simulink model "PBA3_4"  (R2015a)
settings: Solver=ode45  StartTime=0.0  StopTime=18  MaxStep=0.001  MinStep=0.0001  RelTol=1e-3
values from neighbouring files (symbols this model uses):
  c = 0.08    [Bicycle_whipple.m]    (also in PBA3_2_script.m = 0.1; PBA3_4_script.m = 0.1)
  g = 9.81    [Bicycle_whipple.m]    (also in PBA1_script.m; PBA3_2_script.m; PBA3_4_script.m; cruise_control.m)
  K = K0+K2*v0^2    [Bicycle_whipple.m]    (also in PBA3_4_script.m = acker(sys.a, sys.b, P); extended_kalman_filter.m = Ppred(:,:,k+1) * dH'/(R - dH*Ppred(:,:,k+1)*dH'); setup_lab_heli_3d_skeleton_Harry.m = lqr(A, B, Qx, Qu))
  l = 1    [PBA3_2_script.m]    (also in PBA3_4_script.m)
  m = 1200    [PBA1_script.m]    (also in PBA3_2_script.m = 80; PBA3_4_script.m = 80; cruise_control.m = 1000)
  M = [Jxxt -Flx-gamma*Jxzt;-Flx-gamma*Jxzt Fll+2*gamma*Flz+gamma^2*Jzzt]    [Bicycle_whipple.m]    (also in PBA3_2_script.m = 10; PBA3_4_script.m = 10)
  rho = 0.01    [PBA3_2_script.m]    (also in PBA3_4_script.m; helicopter_eom.m = sym('rho(t)'))
settings Model: Creator=Callum  LastModifiedBy=Owner
settings HardwareCC: TargetLongLongMode=on  TargetIntDivRoundTo=Zero  TargetEndianess=LittleEndian  TargetHWDeviceType=MATLAB Host  ProdEqTarget=off
settings RTWCC: SystemTargetFile=rsim.tlc  TemplateMakefile=rsim_default_tmf  Description=Rapid Simulation Target
settings RSimTargetCC: ERTMultiwordTypeDef=System defined  ERTMultiwordLength=256

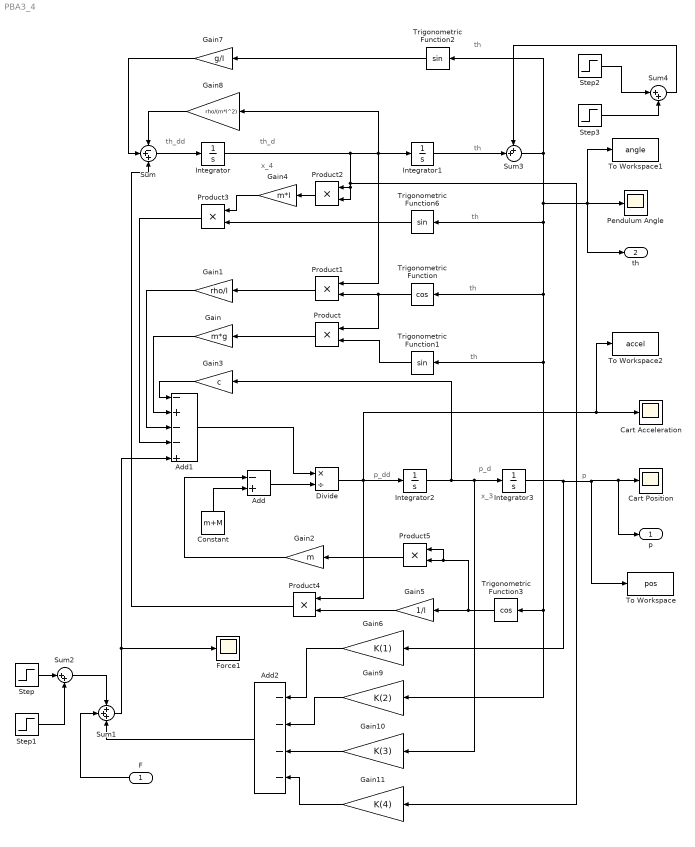
== system PBA3_4 ==
  note: x_4
  note: x_3
  note: th
  note: th
  note: th
  note: th
  note: th
  note: th_d
  note: th_dd
  note: p
  note: p_d
  note: p_dd
  F : Inport
  Add : Sum  Inputs=-+
  Add1 : Sum  Inputs=-+--+
  Add2 : Sum  Inputs=----
  Cart Acceleration : Scope
      settings: SaveName=ScopeData2
  Cart Position : Scope
  Constant : Constant  Value=m+M
  Divide : Product  Inputs=*/
  Force1 : Scope
      settings: SaveName=ScopeData3
  Gain : Gain  Gain=m*g
  Gain1 : Gain  Gain=rho/l
  Gain10 : Gain  Gain=K(3)
  Gain11 : Gain  Gain=K(4)
  Gain2 : Gain  Gain=m
  Gain3 : Gain  Gain=c
  Gain4 : Gain  Gain=m*l
  Gain5 : Gain  Gain=1/l
  Gain6 : Gain  Gain=K(1)
  Gain7 : Gain  Gain=g/l
  Gain8 : Gain  Gain=rho/(m*l^2)
  Gain9 : Gain  Gain=K(2)
  Integrator{,1..3} (4 alike) : Integrator
  Pendulum Angle : Scope
  Product{,1..5} (6 alike) : Product
  Step : Step  Time=2  After=70  SampleTime=0
  Step1 : Step  Time=3  After=-70  SampleTime=0
  Step2 : Step  Time=0  After=pi/2  SampleTime=0
  Step3 : Step  Time=0.01  After=-pi/2  SampleTime=0
  Sum : Sum  Inputs=-++
  Sum1 : Sum  Inputs=+++
  Sum2 : Sum  Inputs=|++
  Sum3 : Sum  Inputs=++|
  Sum4 : Sum  Inputs=|++
  To Workspace : ToWorkspace  VariableName=pos  SaveFormat=Timeseries  SampleTime=-1
  To Workspace1 : ToWorkspace  VariableName=angle  SaveFormat=Timeseries  SampleTime=-1
  To Workspace2 : ToWorkspace  VariableName=accel  SaveFormat=Timeseries  SampleTime=-1
  Trigonometric Function : Trigonometry  Operator=cos
  Trigonometric Function1 : Trigonometry
  Trigonometric Function2 : Trigonometry
  Trigonometric Function3 : Trigonometry  Operator=cos
  Trigonometric Function6 : Trigonometry
  p : Outport
  th : Outport  Port=2
  wires:
  Integrator/1 -> Integrator1/1, Gain8/1, Product1/1, Product2/2, Product2/1, Gain11/1
  Integrator2/1 -> Integrator3/1, Gain10/1, Gain3/1
  Divide/1 -> To Workspace2/1, Cart Acceleration/1, Product4/1, Integrator2/1
  Trigonometric Function/1 -> Product1/2, Product/1
  Trigonometric Function1/1 -> Product/2
  Product/1 -> Gain/1
  Product1/1 -> Gain1/1
  Product5/1 -> Gain2/1
  Add/1 -> Divide/2
  Add1/1 -> Divide/1
  Product2/1 -> Gain4/1
  Gain4/1 -> Product3/1
  Sum/1 -> Integrator/1
  Gain7/1 -> Sum/2
  Integrator3/1 -> Gain6/1, p/1, Cart Position/1, To Workspace/1
  Sum3/1 -> To Workspace1/1, th/1, Pendulum Angle/1, Gain9/1, Trigonometric Function3/1, Trigonometric Function1/1, Trigonometric Function/1, Trigonometric Function6/1, Trigonometric Function2/1
  Trigonometric Function3/1 -> Gain5/1, Product5/1, Product5/2
  Trigonometric Function2/1 -> Gain7/1
  Trigonometric Function6/1 -> Product3/2
  Product4/1 -> Sum/3
  Gain8/1 -> Sum/1
  Sum1/1 -> Add1/5, Force1/1
  Gain3/1 -> Add1/1
  Product3/1 -> Add1/4
  Gain1/1 -> Add1/3
  Gain/1 -> Add1/2
  Gain2/1 -> Add/1
  Constant/1 -> Add/2
  Gain5/1 -> Product4/2
  Gain6/1 -> Add2/1
  Gain9/1 -> Add2/2
  Gain10/1 -> Add2/3
  Gain11/1 -> Add2/4
  Step/1 -> Sum2/1
  Step1/1 -> Sum2/2
  Add2/1 -> Sum1/3
  F/1 -> Sum1/2
  Sum2/1 -> Sum1/1
  Integrator1/1 -> Sum3/2
  Step2/1 -> Sum4/1
  Step3/1 -> Sum4/2
  Sum4/1 -> Sum3/1
